simulink model "Test_Agent_Motor"  (R2018a)
settings: Solver=FixedStepAuto  StartTime=0.0  StopTime=inf  FixedStep=0.000001  RelTol=1e-3
(part 1 of 2)
settings Model: Creator=lenovo  LastModifiedBy=lenovo

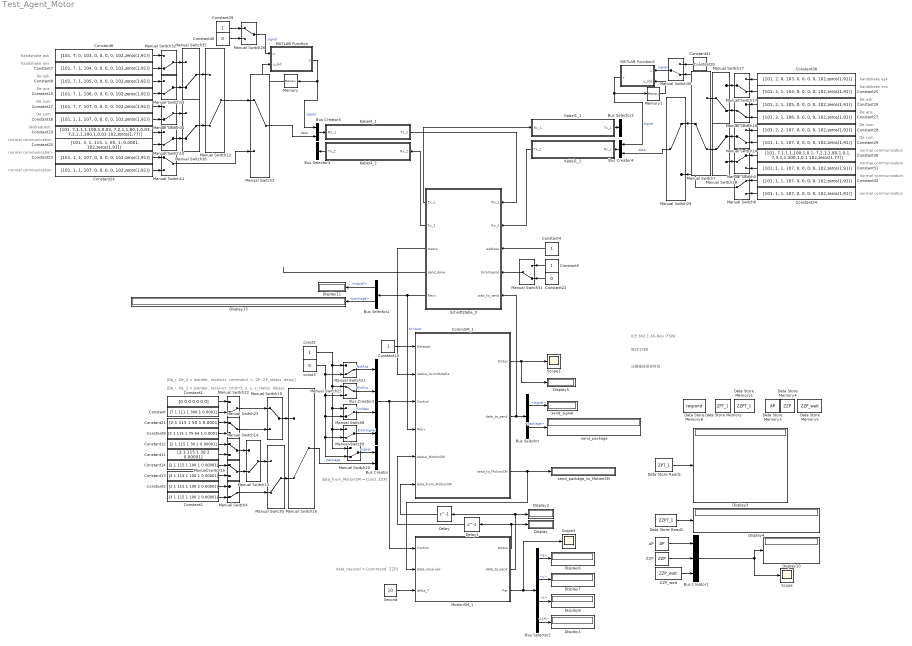
== system Test_Agent_Motor ==
  note: data_reeived = [command, ZZP]
  note: IEEE1588
  note: data_from_MotionSM = [cmd, ZZP]
  note: ICE 802.1 AS-Rev (TSN)
  note: [Da_i, De_i] = [sender, receiver, cmd=5, n, s, s_status, delay]
  note: [Da_i, De_i] = [sender, receiver, command, n, ZP, ZP_status, delay]
  note: 注意修改采样时间
  note: normal communication
  note: normal communication
  note: De ask
  note: handshake ans
  note: De sum
  note: normal communication
  note: handshake ask
  note: normal communication
  note: De sum
  note: normal communication
  note: De sum
  note: normal communication
  note: handshake ans
  note: handshake ask
  note: De ask
  note: Skillrequest
  note: De sum
  note: normal communication
  note: De ans
  note: De ans
  AP : DataStoreRead  DataStoreName=AP
  Bus Creator1 : BusCreator  Inputs=3
  Bus Creator : BusCreator  Inputs=2
  Bus Creator2 : BusCreator  Inputs=4
  Bus Creator4 : BusCreator  Inputs=2
  Bus Creator5 : BusCreator  Inputs=2
  Bus Selector : BusSelector  OutputSignals=signal,package
  Bus Selector1 : BusSelector  OutputSignals=a,v,s,AP
  Bus Selector2 : BusSelector  OutputSignals=signal,package
  Bus Selector3 : BusSelector  OutputSignals=signal,data
  Bus Selector4 : BusSelector  OutputSignals=signal,data
  CommSM_1 : Subsystem
  Constant : Constant  Value=[7 1 111 1 300 1 0.0001]  OutDataTypeStr=double
  Constant1 : Constant  Value=[0 0 0 0 0 0 0]  OutDataTypeStr=double
  Constant10 : Constant  Value=[101, 7, 1, 106, 0, 0, 0, 0, 102,zeros(1,91)]  OutDataTypeStr=double
  Constant11 : Constant  Value=[3 1 115 1 30 2 0.00001]  OutDataTypeStr=double
  Constant12 : Constant  Value=[2 1 115 1 30 2 0.00001]  OutDataTypeStr=double
  Constant13 : Constant  Value=[3 1 115 1 100 1 0.00001]  OutDataTypeStr=double
  Constant14 : Constant  Value=[2 1 115 1 100 1 0.00001]  OutDataTypeStr=double
  Constant15 : Constant  OutDataTypeStr=double
  Constant17 : Constant  Value=[101, 7, 7, 107, 0, 0, 0, 0, 102,zeros(1,91)]  OutDataTypeStr=double
  Constant{18,23..24,29,31..32,34} (7 alike) : Constant  Value=[101, 1, 1, 107, 0, 0, 0, 0, 102,zeros(1,91)]  OutDataTypeStr=double
  Constant19 : Constant  Value=[101, 7,1,1,1,100,1,0.03, 7,2,1,1,80,1,0.03, 7,3,1,1,300,1,0.03 102,zeros(1,77)]  OutDataTypeStr=double
  Constant2 : Constant  Value=[3 1 115 1 100 2 0.00001]  OutDataTypeStr=double
  Constant20 : Constant  Value=[101, 3, 1, 115, 1, 65, 1, 0.0001, 102,zeros(1,91)]  OutDataTypeStr=double
  Constant21 : Constant  Value=[2 1 115 1 50 1 0.0001]  OutDataTypeStr=double
  Constant22 : Constant  Value=0  OutDataTypeStr=boolean
  Constant25 : Constant  Value=[101, 2, 1, 104, 0, 0, 0, 0, 102,zeros(1,91)]  OutDataTypeStr=double
  Constant26 : Constant  Value=[101, 2, 1, 105, 0, 0, 0, 0, 102,zeros(1,91)]  OutDataTypeStr=double
  Constant27 : Constant  Value=[101, 2, 1, 106, 0, 0, 0, 0, 102,zeros(1,91)]  OutDataTypeStr=double
  Constant28 : Constant  Value=[101, 2, 2, 107, 0, 0, 0, 0, 102,zeros(1,91)]  OutDataTypeStr=double
  Constant3 : Constant  Value=[2 1 115 1 100 2 0.00001]  OutDataTypeStr=double
  Constant30 : Constant  Value=[101, 7,1,1,1,100,1,0.1, 7,2,1,1,80,1,0.1, 7,3,1,1,300,1,0.1 102,zeros(1,77)]  OutDataTypeStr=double
  Constant35 : Constant  Value=0  OutDataTypeStr=boolean
  Constant38 : Constant  Value=[101, 2, 0, 103, 0, 0, 0, 0, 102,zeros(1,91)]  OutDataTypeStr=double
  Constant39 : Constant  OutDataTypeStr=boolean
  Constant4 : Constant  OutDataTypeStr=double
  Constant40 : Constant  Value=0  OutDataTypeStr=boolean
  Constant41 : Constant  OutDataTypeStr=boolean
  Constant5 : Constant  OutDataTypeStr=boolean
  Constant6 : Constant  Value=[101, 7, 0, 103, 0, 0, 0, 0, 102,zeros(1,91)]  OutDataTypeStr=double
  Constant7 : Constant  Value=[101, 7, 1, 104, 0, 0, 0, 0, 102,zeros(1,91)]  OutDataTypeStr=double
  Constant8 : Constant  Value=[101, 7, 1, 105, 0, 0, 0, 0, 102,zeros(1,91)]  OutDataTypeStr=double
  Constant9 : Constant  Value=[3 1 115 1 75.64 1 0.0001]  OutDataTypeStr=double
  Data Store Memory : DataStoreMemory  DataStoreName=ZPT_1  ReadBeforeWriteMsg=warning  WriteAfterWriteMsg=warning  WriteAfterReadMsg=warning  InitialValue=zeros(10,3)  VectorParams1D=off  ShowAdditionalParam=off  OutDataTypeStr=double  Dimensions=[10,3]
  Data Store Memory1 : DataStoreMemory  DataStoreName=ZZPT_1  ReadBeforeWriteMsg=warning  WriteAfterWriteMsg=warning  WriteAfterReadMsg=warning  InitialValue=zeros(3,4)  VectorParams1D=off  ShowAdditionalParam=off  OutDataTypeStr=double  Dimensions=[3,4]
  Data Store Memory3 : DataStoreMemory  DataStoreName=AP  ReadBeforeWriteMsg=warning  WriteAfterWriteMsg=warning  WriteAfterReadMsg=warning  ShowAdditionalParam=off  OutMin=[0]  OutMax=[100]  OutDataTypeStr=double  Dimensions=1
  Data Store Memory4 : DataStoreMemory  DataStoreName=ZZP  ReadBeforeWriteMsg=warning  WriteAfterWriteMsg=warning  WriteAfterReadMsg=warning  ShowAdditionalParam=off  OutDataTypeStr=double  Dimensions=1
  Data Store Memory5 : DataStoreMemory  DataStoreName=ZZP_wait  ReadBeforeWriteMsg=warning  WriteAfterWriteMsg=warning  WriteAfterReadMsg=warning  ShowAdditionalParam=off  OutDataTypeStr=double  Dimensions=1
  Data Store Memory6 : DataStoreMemory  DataStoreName=respond  ReadBeforeWriteMsg=warning  WriteAfterWriteMsg=warning  WriteAfterReadMsg=warning  InitialValue=false  ShowAdditionalParam=off  OutDataTypeStr=boolean  Dimensions=1
  Data Store Read1 : DataStoreRead  DataStoreName=ZPT_1
  Data Store Read2 : DataStoreRead  DataStoreName=ZZPT_1
  Delay : Delay  DelayLength=1
  Delay1 : Delay  DelayLength=1
  Display{,1..8,10..11,13} (12 alike) : Display
      Display1 settings: Format=decimal (Stored Integer)
      Display10 settings: Format=decimal (Stored Integer)
      Display13 settings: Decimation=7
      Display8 settings: Format=decimal (Stored Integer)
  Kabel1_1 : Subsystem  TreatAsAtomicUnit=on
  Kabel1_2 : Subsystem  TreatAsAtomicUnit=on
  Kabel4_1 : Subsystem  TreatAsAtomicUnit=on
  Kabel4_2 : Subsystem  TreatAsAtomicUnit=on
  MATLAB Function : MATLAB Function  TreatAsAtomicUnit=on  SystemSampleTime=0.00001
  MATLAB Function1 : MATLAB Function  TreatAsAtomicUnit=on  SystemSampleTime=0.00001
  Manual Switch{4..5,7..10,12..13,16..18,20..22,24,27,30..36} (23 alike) : ManualSwitch  CurrentSetting=0
  Manual Switch{2..3,6,11,14..15,19,23,25..26,28..29} (12 alike) : ManualSwitch
  Memory : Memory  InitialCondition=false
  Memory1 : Memory  InitialCondition=false
  MotionSM_1 : Subsystem
  Schnittstelle_0 : Subsystem
  Scope : Scope
  Scope1 : Scope
  Scope3 : Scope
  Second : Constant  Value=10
  ZZP : DataStoreRead  DataStoreName=ZZP
  ZZP_wait : DataStoreRead  DataStoreName=ZZP_wait
  const2 : Constant  OutDataTypeStr=boolean
  const3 : Constant  Value=0  OutDataTypeStr=boolean
  send_package : Display
  send_package_to_MotionSM : Display
  send_signal : Display
  wires:
  Bus Selector1/2 -> Display7/1  "<v>"
  Manual Switch14/1 -> Manual Switch13/1
  Constant11/1 -> Manual Switch14/2
  Manual Switch9/1 -> Bus Creator2/4  "ErrorSignal"
  Manual Switch16/1 -> Bus Creator/2  "package"
  Manual Switch21/1 -> Bus Creator2/1  "NotAus"
  Bus Creator2/1 -> MotionSM_1/1(Control), CommSM_1/3(Control)
  CommSM_1/1(status) -> Display5/1, Scope1/1
  ZZP/1 -> Bus Creator1/2
  Manual Switch15/1 -> Manual Switch13/2
  Bus Selector1/3 -> Display8/1  "<s>"
  AP/1 -> Bus Creator1/1
  Manual Switch23/1 -> Manual Switch19/2
  Constant21/1 -> Manual Switch23/1
  Second/1 -> MotionSM_1/3(delta_T)
  ZZP_wait/1 -> Bus Creator1/3
  Manual Switch25/1 -> Bus Creator2/2  "EinAus"
  MotionSM_1/3(Par) -> Scope3/1, Bus Selector1/1
  Manual Switch4/1 -> Manual Switch5/2
  Manual Switch13/1 -> Manual Switch5/1
  Bus Creator1/1 -> Display10/1, Scope/1
  Constant12/1 -> Manual Switch14/1
  Manual Switch20/1 -> Bus Creator/1  "signal"
  MotionSM_1/2(data_to_send) -> Delay/1, Display2/1
  const2/1 -> Manual Switch20/1, Manual Switch9/1, Manual Switch8/1, Manual Switch25/1, Manual Switch21/1
  Delay/1 -> CommSM_1/6(data_from_MotionSM)
  Manual Switch19/1 -> Manual Switch16/1
  Constant13/1 -> Manual Switch15/2
  Constant1/1 -> Manual Switch22/1
  Bus Selector1/1 -> Display6/1  "<a>"
  CommSM_1/3(send_to_MotionSM) -> send_package_to_MotionSM/1, MotionSM_1/2(data_received)
  CommSM_1/2(data_to_send) -> Bus Selector/1, Schnittstelle_0/5(wait_to_send)
  Manual Switch8/1 -> Bus Creator2/3  "Richten"
  Manual Switch22/1 -> Manual Switch19/1
  Constant/1 -> Manual Switch22/2
  Constant9/1 -> Manual Switch23/2
  Bus Selector/2 -> send_package/1  "<package>"
  Bus Selector/1 -> send_signal/1  "<signal>"
  Data Store Read1/1 -> Display3/1
  MotionSM_1/1(status) -> Display/1, Delay1/1
  Delay1/1 -> CommSM_1/5(status_MotionSM)
  Constant2/1 -> Manual Switch4/2
  const3/1 -> Manual Switch20/2, Manual Switch9/2, Manual Switch8/2, Manual Switch25/2, Manual Switch21/2
  Constant3/1 -> Manual Switch4/1
  Manual Switch5/1 -> Manual Switch16/2
  Constant14/1 -> Manual Switch15/1
  Data Store Read2/1 -> Display4/1
  Bus Selector1/4 -> Display1/1  "<AP>"
  Constant35/1 -> Manual Switch30/2
  Manual Switch18/1 -> Manual Switch27/2
  Manual Switch30/1 -> MATLAB Function1/1(u)  "signal"
  Constant17/1 -> Manual Switch34/1
  Manual Switch32/1 -> Manual Switch35/1
  Constant41/1 -> Manual Switch30/1
  Manual Switch24/1 -> Manual Switch28/1
  Constant32/1 -> Manual Switch6/1
  Schnittstelle_0/1(Tx_1) -> Kabel1_1/1(Rx_1)
  Manual Switch26/1 -> MATLAB Function/1(u)  "signal"
  Manual Switch7/1 -> Manual Switch29/1
  Constant29/1 -> Manual Switch24/2
  Memory1/1 -> MATLAB Function1/2(u_old)
  Manual Switch6/1 -> Manual Switch29/2
  Constant6/1 -> Manual Switch32/1
  Manual Switch27/1 -> Manual Switch7/1
  Constant26/1 -> Manual Switch18/1
  Manual Switch17/1 -> Manual Switch27/1
  Constant27/1 -> Manual Switch18/2
  Constant7/1 -> Manual Switch32/2
  MATLAB Function/1(y) -> Bus Creator5/1, Memory/1  "signal"
  Schnittstelle_0/5(Recv) -> CommSM_1/4(Recv), Bus Selector2/1  "to Host"
  Memory/1 -> MATLAB Function/2(u_old)
  Manual Switch29/1 -> Bus Creator4/2  "data"
  Bus Creator4/1 -> Kabel1_2/1(Rx_2)
  Constant38/1 -> Manual Switch17/1
  Constant24/1 -> Manual Switch11/2
  Manual Switch34/1 -> Manual Switch36/1
  Constant10/1 -> Manual Switch33/2
  Constant23/1 -> Manual Switch11/1
  Manual Switch28/1 -> Manual Switch7/2
  Constant5/1 -> Manual Switch31/1
  Manual Switch36/1 -> Manual Switch12/2
  Constant19/1 -> Manual Switch10/1
  Manual Switch3/1 -> Manual Switch28/2
  Constant30/1 -> Manual Switch3/1
  Constant20/1 -> Manual Switch10/2
  Schnittstelle_0/3(status) -> CommSM_1/2(status_Schnittstelle)
  Bus Creator5/1 -> Kabel4_1/1(Rx_1)
  Manual Switch12/1 -> Manual Switch2/1
  Schnittstelle_0/2(Tx_2) -> Kabel4_2/1(Rx_2)
  Manual Switch2/1 -> Bus Creator5/2  "data"
  Constant39/1 -> Manual Switch26/1
  Constant18/1 -> Manual Switch34/2
  Manual Switch33/1 -> Manual Switch35/2
  Manual Switch11/1 -> Manual Switch2/2
  Kabel1_2/1(Tx_2) -> Schnittstelle_0/2(Rx_2)
  MATLAB Function1/1(y) -> Bus Creator4/1, Memory1/1  "signal"
  Constant22/1 -> Manual Switch31/2
  Kabel4_2/1(Tx_2) -> Bus Selector4/1
  Manual Switch31/1 -> Schnittstelle_0/4(ErrorSignal)
  Constant31/1 -> Manual Switch3/2
  Constant8/1 -> Manual Switch33/1
  Kabel1_1/1(Tx_1) -> Bus Selector3/1
  Bus Selector2/2 -> Display13/1  "<package>"
  Bus Selector2/1 -> Display11/1  "<signal>"
  Constant40/1 -> Manual Switch26/2
  Manual Switch35/1 -> Manual Switch12/1
  Manual Switch10/1 -> Manual Switch36/2
  Constant34/1 -> Manual Switch6/2
  Kabel4_1/1(Tx_1) -> Schnittstelle_0/1(Rx_1)
  Constant25/1 -> Manual Switch17/2
  Constant28/1 -> Manual Switch24/1
  Constant4/1 -> Schnittstelle_0/3(address)
  Constant15/1 -> CommSM_1/1(Adresse)
  Schnittstelle_0/4(send_done) -> ?

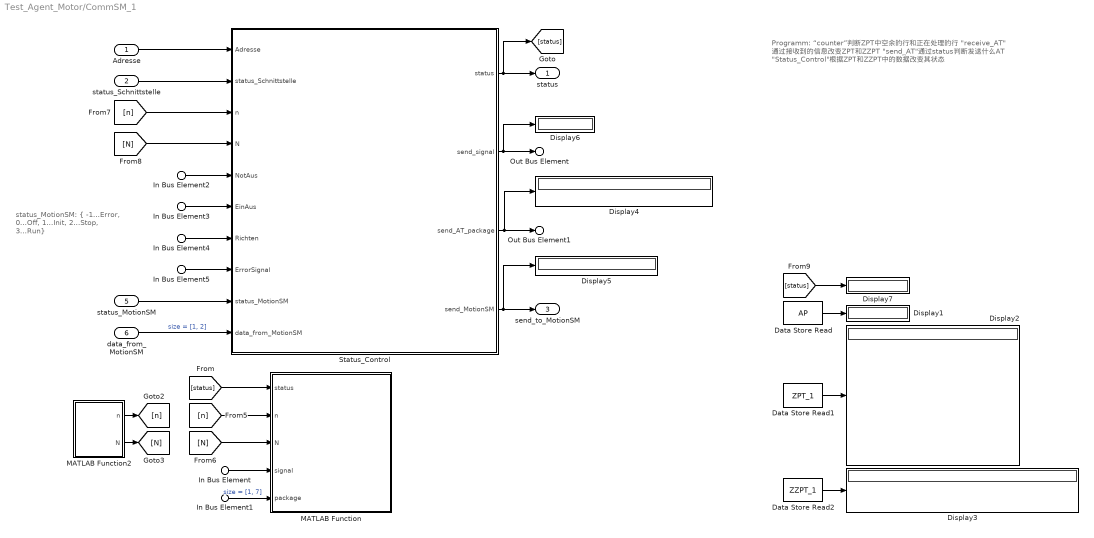
== system Test_Agent_Motor/CommSM_1 ==
  note: Programm:
      | “counter”判断ZPT中空余的行和正在处理的行
      | "receive_AT" 通过接收到的信息改变ZPT和ZZPT
      | "send_AT"通过status判断发送什么AT
      | "Status_Control"根据ZPT和ZZPT中的数据改变其状态
  note: status_MotionSM: {
      | -1...Error,
      | 0...Off,
      | 1...Init,
      | 2...Stop,
      | 3...Run}
  Adresse : Inport  OutDataTypeStr=double  PortDimensions=1
  status_Schnittstelle : Inport  Port=2  OutDataTypeStr=double  PortDimensions=1
  In Bus Element2 : Inport  Port=3  PortName=Control  Element=NotAus
  In Bus Element3 : Inport  Port=3  PortName=Control  Element=EinAus
  In Bus Element4 : Inport  Port=3  PortName=Control  Element=Richten
  In Bus Element5 : Inport  Port=3  PortName=Control  Element=ErrorSignal
  In Bus Element : Inport  Port=4  PortName=Recv  Element=signal
  In Bus Element1 : Inport  Port=4  PortName=Recv  Element=package
  status_MotionSM : Inport  Port=5  OutDataTypeStr=double  PortDimensions=1
  data_from_MotionSM : Inport  Port=6  OutDataTypeStr=double  PortDimensions=2
  Data Store Read : DataStoreRead  DataStoreName=AP
  Data Store Read1 : DataStoreRead  DataStoreName=ZPT_1
  Data Store Read2 : DataStoreRead  DataStoreName=ZZPT_1
  Display{1..7} (7 alike) : Display
  MATLAB Function : MATLAB Function  TreatAsAtomicUnit=on
  MATLAB Function2 : MATLAB Function  TreatAsAtomicUnit=on
  Status_Control : Stateflow chart  TreatAsAtomicUnit=on
  status : Outport  OutDataTypeStr=double  PortDimensions=1
  Out Bus Element : Outport  Port=2  PortName=data_to_send  Element=signal
  Out Bus Element1 : Outport  Port=2  PortName=data_to_send  Element=package
  send_to_MotionSM : Outport  Port=3
  wires:
  In Bus Element2/1 -> Status_Control/5(NotAus)
  In Bus Element3/1 -> Status_Control/6(EinAus)
  In Bus Element4/1 -> Status_Control/7(Richten)
  In Bus Element5/1 -> Status_Control/8(ErrorSignal)
  status_Schnittstelle/1 -> Status_Control/2(status_Schnittstelle)
  In Bus Element/1 -> MATLAB Function/4(signal)
  In Bus Element1/1 -> MATLAB Function/5(package)  "size = [1, 7]"
  data_from_MotionSM/1 -> Status_Control/10(data_from_MotionSM)  "size = [1, 2]"
  status_MotionSM/1 -> Status_Control/9(status_MotionSM)
  Adresse/1 -> Status_Control/1(Adresse)
  Status_Control/1(status) -> [status], status/1
  Status_Control/3(send_AT_package) -> Out Bus Element1/1, Display4/1
  Status_Control/4(send_MotionSM) -> send_to_MotionSM/1, Display5/1
  Status_Control/2(send_signal) -> Out Bus Element/1, Display6/1
  Data Store Read/1 -> Display1/1
  Data Store Read1/1 -> Display2/1
  Data Store Read2/1 -> Display3/1
  [status] -> MATLAB Function/1(status)
  MATLAB Function2/1(n) -> [n]
  MATLAB Function2/2(N) -> [N]
  [N] -> MATLAB Function/3(N)
  [n] -> MATLAB Function/2(n)
  [n] -> Status_Control/3(n)
  [N] -> Status_Control/4(N)
  [status] -> Display7/1

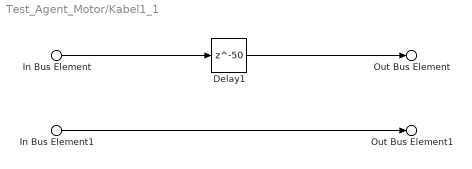
== system Test_Agent_Motor/Kabel1_1 ==
  In Bus Element : Inport  PortName=Rx_1  Element=signal
  In Bus Element1 : Inport  PortName=Rx_1  Element=data
  Delay1 : Delay  DelayLength=50
  Out Bus Element : Outport  PortName=Tx_1  Element=signal
  Out Bus Element1 : Outport  PortName=Tx_1  Element=data
  wires:
  In Bus Element/1 -> Delay1/1
  Delay1/1 -> Out Bus Element/1
  In Bus Element1/1 -> Out Bus Element1/1

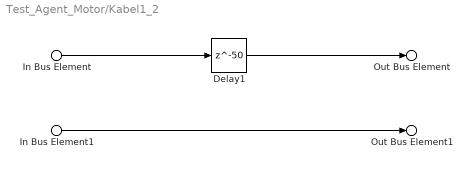
== system Test_Agent_Motor/Kabel1_2 ==
  In Bus Element : Inport  PortName=Rx_2  Element=signal
  In Bus Element1 : Inport  PortName=Rx_2  Element=data
  Delay1 : Delay  DelayLength=50
  Out Bus Element : Outport  PortName=Tx_2  Element=signal
  Out Bus Element1 : Outport  PortName=Tx_2  Element=data
  wires:
  In Bus Element/1 -> Delay1/1
  Delay1/1 -> Out Bus Element/1
  In Bus Element1/1 -> Out Bus Element1/1

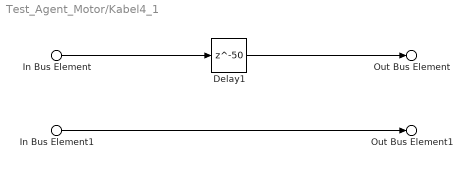
== system Test_Agent_Motor/Kabel4_1 ==
  In Bus Element : Inport  PortName=Rx_1  Element=signal
  In Bus Element1 : Inport  PortName=Rx_1  Element=data
  Delay1 : Delay  DelayLength=50
  Out Bus Element : Outport  PortName=Tx_1  Element=signal
  Out Bus Element1 : Outport  PortName=Tx_1  Element=data
  wires:
  In Bus Element/1 -> Delay1/1
  Delay1/1 -> Out Bus Element/1
  In Bus Element1/1 -> Out Bus Element1/1

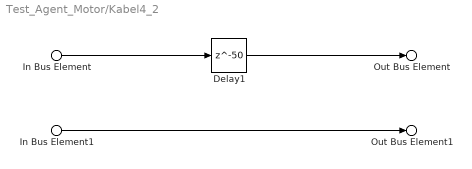
== system Test_Agent_Motor/Kabel4_2 ==
  In Bus Element : Inport  PortName=Rx_2  Element=signal
  In Bus Element1 : Inport  PortName=Rx_2  Element=data
  Delay1 : Delay  DelayLength=50
  Out Bus Element : Outport  PortName=Tx_2  Element=signal
  Out Bus Element1 : Outport  PortName=Tx_2  Element=data
  wires:
  In Bus Element/1 -> Delay1/1
  Delay1/1 -> Out Bus Element/1
  In Bus Element1/1 -> Out Bus Element1/1

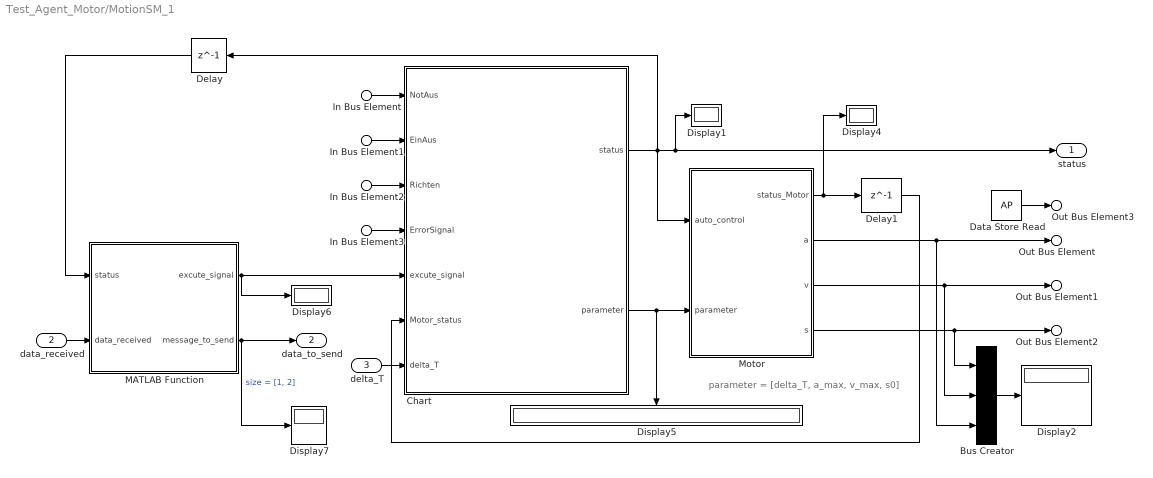
== system Test_Agent_Motor/MotionSM_1 ==
  note: parameter = [delta_T, a_max, v_max, s0]
  In Bus Element : Inport  PortName=Control  Element=NotAus
  In Bus Element1 : Inport  PortName=Control  Element=EinAus
  In Bus Element2 : Inport  PortName=Control  Element=Richten
  In Bus Element3 : Inport  PortName=Control  Element=ErrorSignal
  data_received : Inport  Port=2  OutDataTypeStr=double  PortDimensions=2
  delta_T : Inport  Port=3
  Bus Creator : BusCreator  Inputs=3
  Chart : Stateflow chart  TreatAsAtomicUnit=on
  Data Store Read : DataStoreRead  DataStoreName=AP
  Delay : Delay  DelayLength=1
  Delay1 : Delay  DelayLength=1
  Display{1..2,4..7} (6 alike) : Display
  MATLAB Function : MATLAB Function  TreatAsAtomicUnit=on
  Motor : Subsystem
  status : Outport
  data_to_send : Outport  Port=2  OutDataTypeStr=double  PortDimensions=2
  Out Bus Element : Outport  Port=3  PortName=Par  Element=a
  Out Bus Element1 : Outport  Port=3  PortName=Par  Element=v
  Out Bus Element2 : Outport  Port=3  PortName=Par  Element=s
  Out Bus Element3 : Outport  Port=3  PortName=Par  Element=AP
  wires:
  Chart/1(status) -> Motor/1(auto_control), Delay/1, Display1/1, status/1
  In Bus Element1/1 -> Chart/2(EinAus)
  In Bus Element/1 -> Chart/1(NotAus)
  In Bus Element2/1 -> Chart/3(Richten)
  In Bus Element3/1 -> Chart/4(ErrorSignal)
  Motor/1(status_Motor) -> Display4/1, Delay1/1
  data_received/1 -> MATLAB Function/2(data_received)
  Delay1/1 -> Chart/6(Motor_status)
  MATLAB Function/1(excute_signal) -> Display6/1, Chart/5(excute_signal)
  MATLAB Function/2(message_to_send) -> data_to_send/1, Display7/1  "size = [1, 2]"
  delta_T/1 -> Chart/7(delta_T)
  Motor/2(a) -> Bus Creator/3, Out Bus Element/1
  Motor/3(v) -> Bus Creator/2, Out Bus Element1/1
  Motor/4(s) -> Bus Creator/1, Out Bus Element2/1
  Chart/2(parameter) -> Motor/2(parameter), Display5/1
  Delay/1 -> MATLAB Function/1(status)
  Data Store Read/1 -> Out Bus Element3/1
  Bus Creator/1 -> Display2/1

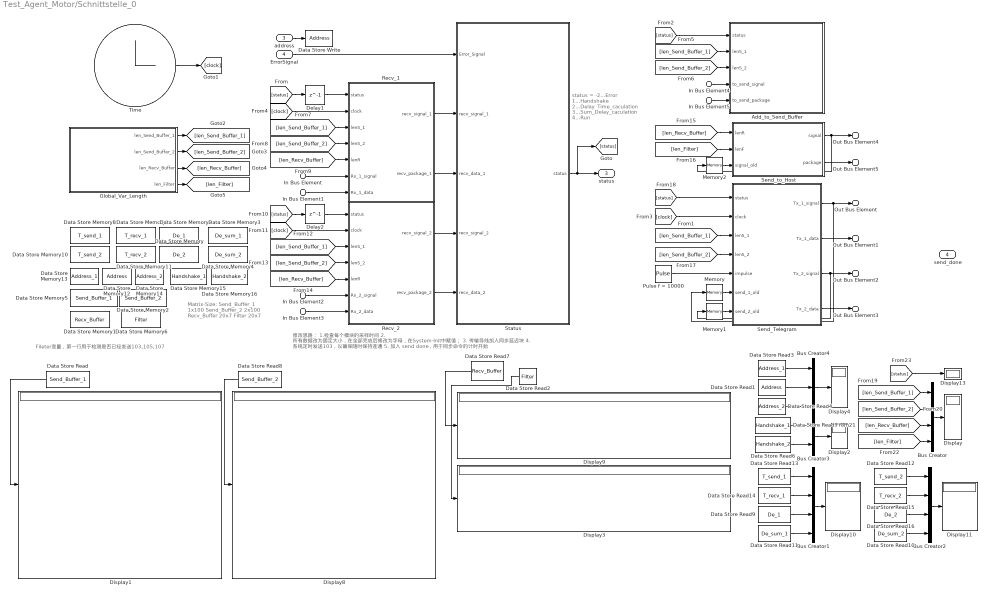
== system Test_Agent_Motor/Schnittstelle_0 ==
  note: Fileter变量，第一行用于检测是否已经发送103,105,107
  note: 修改思路：
      | 1.检查每个模块的采样时间
      | 2. 所有数据改为固定大小，在全部完成后修改为字母，在System-Init中赋值；
      | 3. 传输导线加入同步延迟块
      | 4. 系统定时发送103，以确保随时保持连通
      | 5. 加入 send done，用于同步命令的计时开始
  note: status =
      | -2...Error
      |  1...Handshake
      |  2...Delay_Time_caculation
      |  3...Sum_Delay_caculation
      |  4...Run
  note: Matrix-Size:
      | Send_Buffer_1	1x100
      | Send_Buffer_2	2x100
      | Recv_Buffer		20x7
      | Filter			20x7
  In Bus Element : Inport  PortName=Rx_1  Element=signal
  In Bus Element1 : Inport  PortName=Rx_1  Element=data
  In Bus Element2 : Inport  Port=2  PortName=Rx_2  Element=signal
  In Bus Element3 : Inport  Port=2  PortName=Rx_2  Element=data
  address : Inport  Port=3
  ErrorSignal : Inport  Port=4
  In Bus Element4 : Inport  Port=5  PortName=wait_to_send  Element=signal
  In Bus Element5 : Inport  Port=5  PortName=wait_to_send  Element=package
  Add_to_Send_Buffer : MATLAB Function  TreatAsAtomicUnit=on  SystemSampleTime=0.00001
  Bus Creator : BusCreator  Inputs=4
  Bus Creator1 : BusCreator  Inputs=4
  Bus Creator2 : BusCreator  Inputs=4
  Bus Creator3 : BusCreator  Inputs=2
  Bus Creator4 : BusCreator  Inputs=3
  Data Store Memory : DataStoreMemory  DataStoreName=De_2  ReadBeforeWriteMsg=warning  WriteAfterWriteMsg=warning  WriteAfterReadMsg=warning  ShowAdditionalParam=off  OutDataTypeStr=double  Dimensions=1
  Data Store Memory1 : DataStoreMemory  DataStoreName=Recv_Buffer  ReadBeforeWriteMsg=warning  WriteAfterWriteMsg=warning  WriteAfterReadMsg=warning  InitialValue=zeros(20,7)  VectorParams1D=off  ShowAdditionalParam=off  OutDataTypeStr=double  Dimensions=[20,7]
  Data Store Memory10 : DataStoreMemory  DataStoreName=T_send_2  ReadBeforeWriteMsg=warning  WriteAfterWriteMsg=warning  WriteAfterReadMsg=warning  ShowAdditionalParam=off  OutDataTypeStr=double  Dimensions=1
  Data Store Memory11 : DataStoreMemory  DataStoreName=T_recv_2  ReadBeforeWriteMsg=warning  WriteAfterWriteMsg=warning  WriteAfterReadMsg=warning  ShowAdditionalParam=off  OutDataTypeStr=double  Dimensions=1
  Data Store Memory12 : DataStoreMemory  DataStoreName=Address  ReadBeforeWriteMsg=warning  WriteAfterWriteMsg=warning  WriteAfterReadMsg=warning  ShowAdditionalParam=off  OutDataTypeStr=double  Dimensions=1
  Data Store Memory13 : DataStoreMemory  DataStoreName=Address_1  ReadBeforeWriteMsg=warning  WriteAfterWriteMsg=warning  WriteAfterReadMsg=warning  ShowAdditionalParam=off  OutDataTypeStr=double  Dimensions=1
  Data Store Memory14 : DataStoreMemory  DataStoreName=Address_2  ReadBeforeWriteMsg=warning  WriteAfterWriteMsg=warning  WriteAfterReadMsg=warning  ShowAdditionalParam=off  OutDataTypeStr=double  Dimensions=1
  Data Store Memory15 : DataStoreMemory  DataStoreName=Handshake_1  ReadBeforeWriteMsg=warning  WriteAfterWriteMsg=warning  WriteAfterReadMsg=warning  InitialValue=false  ShowAdditionalParam=off  OutDataTypeStr=boolean
  Data Store Memory16 : DataStoreMemory  DataStoreName=Handshake_2  ReadBeforeWriteMsg=warning  WriteAfterWriteMsg=warning  WriteAfterReadMsg=warning  InitialValue=false  ShowAdditionalParam=off  OutDataTypeStr=boolean
  Data Store Memory2 : DataStoreMemory  DataStoreName=Send_Buffer_2  ReadBeforeWriteMsg=warning  WriteAfterWriteMsg=warning  WriteAfterReadMsg=warning  InitialValue=[101, 102, zeros(1,98)]  VectorParams1D=off  ShowAdditionalParam=off  OutDataTypeStr=double  Dimensions=[1,100]
  Data Store Memory3 : DataStoreMemory  DataStoreName=De_sum_1  ReadBeforeWriteMsg=warning  WriteAfterWriteMsg=warning  WriteAfterReadMsg=warning  ShowAdditionalParam=off  OutDataTypeStr=double  Dimensions=1
  Data Store Memory4 : DataStoreMemory  DataStoreName=De_sum_2  ReadBeforeWriteMsg=warning  WriteAfterWriteMsg=warning  WriteAfterReadMsg=warning  ShowAdditionalParam=off  OutDataTypeStr=double  Dimensions=1
  Data Store Memory5 : DataStoreMemory  DataStoreName=Send_Buffer_1  ReadBeforeWriteMsg=warning  WriteAfterWriteMsg=warning  WriteAfterReadMsg=warning  InitialValue=[101, 102, zeros(1,98)]  VectorParams1D=off  ShowAdditionalParam=off  OutDataTypeStr=double  Dimensions=[1,100]
  Data Store Memory6 : DataStoreMemory  DataStoreName=Filter  ReadBeforeWriteMsg=warning  WriteAfterWriteMsg=warning  WriteAfterReadMsg=warning  InitialValue=zeros(20,7)  VectorParams1D=off  ShowAdditionalParam=off  OutDataTypeStr=double  Dimensions=[20,7]
  Data Store Memory7 : DataStoreMemory  DataStoreName=De_1  ReadBeforeWriteMsg=warning  WriteAfterWriteMsg=warning  WriteAfterReadMsg=warning  ShowAdditionalParam=off  OutDataTypeStr=double  Dimensions=1
  Data Store Memory8 : DataStoreMemory  DataStoreName=T_send_1  ReadBeforeWriteMsg=warning  WriteAfterWriteMsg=warning  WriteAfterReadMsg=warning  ShowAdditionalParam=off  OutDataTypeStr=double  Dimensions=1
  Data Store Memory9 : DataStoreMemory  DataStoreName=T_recv_1  ReadBeforeWriteMsg=warning  WriteAfterWriteMsg=warning  WriteAfterReadMsg=warning  ShowAdditionalParam=off  OutDataTypeStr=double  Dimensions=1
  Data Store Read : DataStoreRead  DataStoreName=Send_Buffer_1
  Data Store Read1 : DataStoreRead  DataStoreName=Address
  Data Store Read10 : DataStoreRead  DataStoreName=De_sum_2
  Data Store Read11 : DataStoreRead  DataStoreName=De_sum_1
  Data Store Read12 : DataStoreRead  DataStoreName=T_send_2
  Data Store Read13 : DataStoreRead  DataStoreName=T_send_1
  Data Store Read14 : DataStoreRead  DataStoreName=T_recv_1
  Data Store Read15 : DataStoreRead  DataStoreName=T_recv_2
  Data Store Read16 : DataStoreRead  DataStoreName=De_2
  Data Store Read2 : DataStoreRead  DataStoreName=Filter
  Data Store Read3 : DataStoreRead  DataStoreName=Address_1
  Data Store Read4 : DataStoreRead  DataStoreName=Address_2
  Data Store Read5 : DataStoreRead  DataStoreName=Handshake_1
  Data Store Read6 : DataStoreRead  DataStoreName=Handshake_2
  Data Store Read7 : DataStoreRead  DataStoreName=Recv_Buffer
  Data Store Read8 : DataStoreRead  DataStoreName=Send_Buffer_2
  Data Store Read9 : DataStoreRead  DataStoreName=De_1
  Data Store Write : DataStoreWrite  DataStoreName=Address
  Delay1 : Delay  DelayLength=1
  Delay2 : Delay  DelayLength=1
  Display{,1..4,8..11,13} (10 alike) : Display
  Global_Var_Length : MATLAB Function  TreatAsAtomicUnit=on
  Memory : Memory  InitialCondition=false
  Memory1 : Memory  InitialCondition=false
  Memory2 : Memory  InitialCondition=false
  Pulse f = 10000 : DiscretePulseGenerator  PulseType=Time based  Amplitude=true  Period=1/1000  PulseWidth=30
  Recv_1 : MATLAB Function  TreatAsAtomicUnit=on  SystemSampleTime=0.00001
  Recv_2 : MATLAB Function  TreatAsAtomicUnit=on  SystemSampleTime=0.00001
  Send_Telegram : MATLAB Function  TreatAsAtomicUnit=on  SystemSampleTime=0.00001
  Send_to_Host : MATLAB Function  TreatAsAtomicUnit=on  SystemSampleTime=0.00001
  Status : Stateflow chart  TreatAsAtomicUnit=on  SystemSampleTime=0.0000001
  Time : Clock
  Out Bus Element : Outport  PortName=Tx_1  Element=signal
  Out Bus Element1 : Outport  PortName=Tx_1  Element=data
  Out Bus Element2 : Outport  Port=2  PortName=Tx_2  Element=signal
  Out Bus Element3 : Outport  Port=2  PortName=Tx_2  Element=data
  status : Outport  Port=3
  send_done : Outport  Port=4
  Out Bus Element4 : Outport  Port=5  PortName=Recv  Element=signal
  Out Bus Element5 : Outport  Port=5  PortName=Recv  Element=package
  wires:
  ErrorSignal/1 -> Status/1(Error_Signal)
  Status/1(status) -> [status], status/1
  Pulse f = 10000/1 -> Send_Telegram/5(impulse)
  In Bus Element1/1 -> Recv_1/7(Rx_1_data)
  In Bus Element/1 -> Recv_1/6(Rx_1_signal)
  Send_Telegram/1(Tx_1_signal) -> Memory/1, Out Bus Element/1
  Send_Telegram/3(Tx_2_signal) -> Memory1/1, Out Bus Element2/1
  Memory1/1 -> Send_Telegram/7(send_2_old)
  Memory/1 -> Send_Telegram/6(send_1_old)
  [status] -> Delay1/1
  Time/1 -> [clock]
  [clock] -> Recv_1/2(clock)
  Send_to_Host/1(signal) -> Out Bus Element4/1, Memory2/1
  address/1 -> Data Store Write/1
  Global_Var_Length/1(len_Send_Buffer_1) -> [len_Send_Buffer_1]
  Global_Var_Length/2(len_Send_Buffer_2) -> [len_Send_Buffer_2]
  Global_Var_Length/3(len_Recv_Buffer) -> [len_Recv_Buffer]
  Global_Var_Length/4(len_Filter) -> [len_Filter]
  [len_Send_Buffer_1] -> Recv_1/3(lenS_1)
  [len_Send_Buffer_2] -> Recv_1/4(lenS_2)
  [len_Recv_Buffer] -> Recv_1/5(lenR)
  In Bus Element2/1 -> Recv_2/6(Rx_2_signal)
  In Bus Element3/1 -> Recv_2/7(Rx_2_data)
  [status] -> Delay2/1
  [len_Recv_Buffer] -> Recv_2/5(lenR)
  [len_Send_Buffer_1] -> Recv_2/3(lenS_1)
  [clock] -> Recv_2/2(clock)
  [len_Send_Buffer_2] -> Recv_2/4(lenS_2)
  Delay1/1 -> Recv_1/1(status)
  Delay2/1 -> Recv_2/1(status)
  Recv_1/1(recv_signal_1) -> Status/2(recv_signal_1)
  Recv_1/2(recv_package_1) -> Status/3(recv_data_1)
  Recv_2/1(recv_signal_2) -> Status/4(recv_signal_2)
  Recv_2/2(recv_package_2) -> Status/5(recv_data_2)
  [len_Recv_Buffer] -> Send_to_Host/1(lenR)
  [len_Filter] -> Send_to_Host/2(lenF)
  Send_Telegram/4(Tx_2_data) -> Out Bus Element3/1
  [len_Send_Buffer_1] -> Send_Telegram/3(lenS_1)
  [len_Send_Buffer_2] -> Send_Telegram/4(lenS_2)
  [clock] -> Send_Telegram/2(clock)
  [status] -> Send_Telegram/1(status)
  Send_Telegram/2(Tx_1_data) -> Out Bus Element1/1
  [len_Send_Buffer_1] -> Add_to_Send_Buffer/2(lenS_1)
  [len_Send_Buffer_2] -> Add_to_Send_Buffer/3(lenS_2)
  In Bus Element4/1 -> Add_to_Send_Buffer/4(to_send_signal)
  In Bus Element5/1 -> Add_to_Send_Buffer/5(to_send_package)
  [status] -> Add_to_Send_Buffer/1(status)
  Memory2/1 -> Send_to_Host/3(signal_old)
  Bus Creator/1 -> Display/1
  [len_Send_Buffer_1] -> Bus Creator/1
  [len_Send_Buffer_2] -> Bus Creator/2
  [len_Recv_Buffer] -> Bus Creator/3
  [len_Filter] -> Bus Creator/4
  Data Store Read/1 -> Display1/1
  Data Store Read2/1 -> Display3/1
  Data Store Read8/1 -> Display8/1
  Data Store Read7/1 -> Display9/1
  Data Store Read13/1 -> Bus Creator1/1
  Data Store Read14/1 -> Bus Creator1/2
  Data Store Read11/1 -> Bus Creator1/4
  Data Store Read9/1 -> Bus Creator1/3
  Bus Creator1/1 -> Display10/1
  Data Store Read12/1 -> Bus Creator2/1
  Data Store Read15/1 -> Bus Creator2/2
  Bus Creator2/1 -> Display11/1
  Data Store Read16/1 -> Bus Creator2/3
  Data Store Read10/1 -> Bus Creator2/4
  [status] -> Display13/1
  Send_to_Host/2(package) -> Out Bus Element5/1
  Data Store Read5/1 -> Bus Creator3/1
  Data Store Read6/1 -> Bus Creator3/2
  Data Store Read4/1 -> Bus Creator4/3
  Data Store Read1/1 -> Bus Creator4/2
  Data Store Read3/1 -> Bus Creator4/1
  Bus Creator3/1 -> Display2/1
  Bus Creator4/1 -> Display4/1

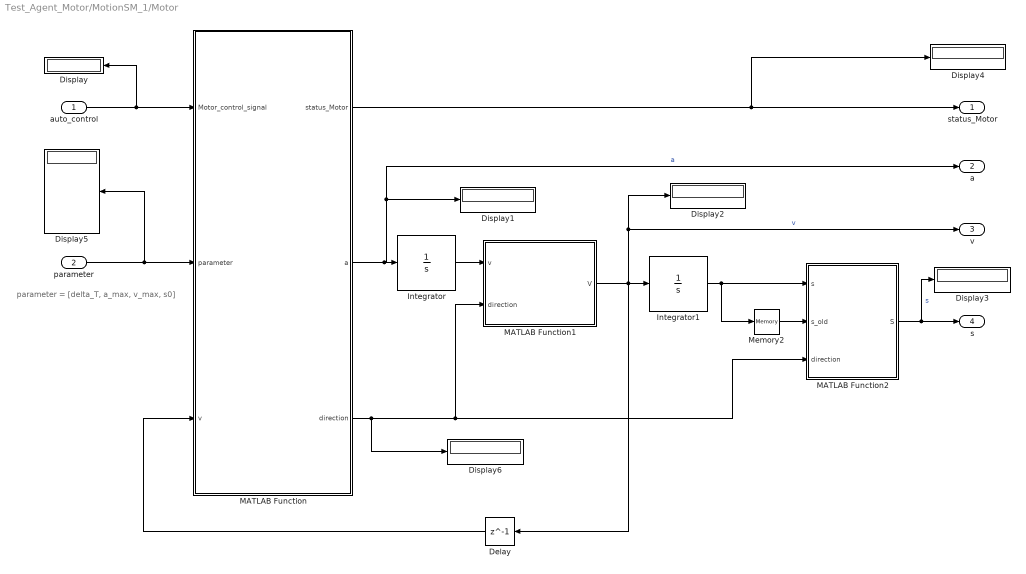
== system Test_Agent_Motor/MotionSM_1/Motor ==
  note: parameter = [delta_T, a_max, v_max, s0]
  auto_control : Inport
  parameter : Inport  Port=2
  Delay : Delay  DelayLength=1
  Display{,1..6} (7 alike) : Display
  Integrator : Integrator
  Integrator1 : Integrator
  MATLAB Function : MATLAB Function  TreatAsAtomicUnit=on
  MATLAB Function1 : MATLAB Function  TreatAsAtomicUnit=on
  MATLAB Function2 : MATLAB Function  TreatAsAtomicUnit=on
  Memory2 : Memory
  status_Motor : Outport
  a : Outport  Port=2
  v : Outport  Port=3
  s : Outport  Port=4
  wires:
  Integrator/1 -> MATLAB Function1/1(v)
  Integrator1/1 -> MATLAB Function2/1(s), Memory2/1
  auto_control/1 -> Display/1, MATLAB Function/1(Motor_control_signal)
  MATLAB Function/1(status_Motor) -> Display4/1, status_Motor/1
  parameter/1 -> Display5/1, MATLAB Function/2(parameter)
  MATLAB Function/2(a) -> a/1, Display1/1, Integrator/1  "a"
  MATLAB Function1/1(V) -> Display2/1, v/1, Delay/1, Integrator1/1  "v"
  MATLAB Function/3(direction) -> MATLAB Function1/2(direction), MATLAB Function2/3(direction), Display6/1
  MATLAB Function2/1(S) -> Display3/1, s/1  "s"
  Memory2/1 -> MATLAB Function2/2(s_old)
  Delay/1 -> MATLAB Function/3(v)

== matlab function Test_Agent_Motor/MotionSM_1/MATLAB Function ==
  data: status input double size=1; excute_signal output boolean size=1; message_to_send output double size=2; data_received input double size=2; ZZP_wait data_store_memory size=1; AP data_store_memory; ZZP data_store_memory
%data_received / message_to_send = [cmd, ZZP]
%cmd:  1...setP, 2...getP, 3...excP

function [excute_signal, message_to_send] = message_analysis(status, data_received)

global ZZP_wait
global AP
global ZZP

excute_signal = false;

cmd = data_received(1);
message_to_send = [0, 0]';

switch cmd
    case 1      % setP
        excute_signal = false;
        if ((status >= 1) && (status <= 3))
            ZZP_wait = data_received(2);
            message_to_send = [2, ZZP_wait]';   % getP
        end
        
    case 3      % excP
        excute_signal = true;
        if ((ZZP == AP) && (status == 2) && (ZZP~=ZZP_wait))
            ZZP = ZZP_wait;
        end
end
end

== matlab function Test_Agent_Motor/MotionSM_1/Motor/MATLAB Function ==
  settings: updateMethod=DISCRETE
  data: status_Motor output boolean size=1; Motor_control_signal input double size=1; parameter input double size=4; v input double size=1; a output double size=1; direction output double size=1; AP data_store_memory; ZZP data_store_memory
function [status_Motor, a, direction]= Motor(Motor_control_signal, parameter, v)

%delta_T = parameter(1);
a_max = abs(parameter(2));
v_max = abs(parameter(3));
s0 = parameter(4);
direction = 0;
a = 0;

s_a = 0.5 * v_max * v_max / a_max;
a_bremsen = 100000;     % 100 m/s^2

global AP
global ZZP

switch Motor_control_signal
    case {-1, 0}            %Error & Off
        if v > 0
            a = -a_bremsen;
            direction = 1;
        elseif v < 0
            a = a_bremsen;
            direction = -1;
        else
            a = 0;
            direction = 0;
        end
             
    case 1                  %Init
        if (AP > 0)
            direction = s0;
            if ((ZZP - AP) < (-s_a)) && (v > (-v_max))
                a = -a_max;
            elseif ((ZZP - AP) >= (-s_a)) && (ZZP < AP) && (v < 0)
                a = a_max;
            else
                a = 0;
            end
        else
            a = 0;
            AP = 0;
        end
        
    case 2                  %Stop
        if (v > 0)
            a = -a_max;
            direction = 1;
        elseif (v < 0)
            a = a_max;
            direction = -1;
        else
            a = 0;
            direction = 0;
        end
        
    case 3                  %run
        direction = s0;
        if (s0 > 0)   %forward
            %v_control(2) = s0;
            if ((ZZP - AP) > s_a) && (v < v_max)
                a = a_max;
            elseif ((ZZP - AP) <= s_a) && (ZZP > AP) && (v > 0)
                a = -a_max;
            else
                a = 0;
            end
        end
        if (s0 < 0)    %backward
            if ((ZZP - AP) < (-s_a)) && (v > (-v_max))
                a = -a_max;
            elseif ((ZZP - AP) >= (-s_a)) && (ZZP < AP) && (v < 0)
                a = a_max;
            else
                a = 0;
            end
        end
end
        
%status_Motor: false...Stopped, true...Running
if (a == 0) && (v == 0)
    status_Motor = false;
else
    status_Motor = true;
end

end

== stateflow chart Test_Agent_Motor/MotionSM_1/Chart ==
  state Off
    entry: status=0;
  state Init
    entry: status=1; parameter=Par_1(delta_T);
  state On
    state Stop
      entry: status=2;
    state Run
      entry: status=3;
    (default) -> Stop
    Stop -> Run : [excute_signal==1 && ZZP~=AP && Motor_status == 0]
        | {parameter=Par(delta_T)}
    Run -> Stop : [ZZP==AP && ~Motor_status]
  state Error
    entry: status=-1;
  (default) -> Off
  Init -> Off [order 1] : [~EinAus]
  Off -> Init [order 2] : [EinAus && ~ NotAus]{parameter=[delta_T,0,0,0]'}
  Init -> Error [order 2] : [Motor_status==-1 || NotAus || ErrorSignal]
  Off -> Error [order 1] : [EinAus && (ErrorSignal || NotAus)]
  Error -> Off [order 1] : [~EinAus]
  On -> Off [order 1] : [~EinAus]
  Error -> Init [order 2] : [Richten]{parameter=[delta_T,0,0,0]'}
  Init -> On [order 3] : [AP==0]{parameter=[delta_T,0,0,0]'}
  On -> Error [order 2] : [Motor_status==-1 || NotAus || ErrorSignal]
  data: par function_output double size=4; delta_t function_input double size=1; par function_output double size=4; delta_t function_input double size=1; NotAus input boolean size=1; EinAus input boolean size=1; Richten input boolean size=1; ErrorSignal input boolean size=1; excute_signal input boolean size=1; Motor_status input boolean size=1; status output double size=1 =0; ZZP data_store_memory; ZZP_wait data_store_memory; parameter output double size=4; AP data_store_memory size=1; delta_T input double size=1
  function par = Par_1(delta_t):
    | function par = Par_1(delta_t)
    | 
    | global ZZP
    | global ZZP_wait
    | global AP
    | 
    | % delta_T = 10 s
    | ZZP = 0;
    | ZZP_wait = 0;
    | s0 = ZZP - AP;
    | a_max = 100;        % 1 m/s^2
    | v_max = 1;
    | %v_max = 0.5 * a_max * (delta_t - sqrt(delta_t*delta_t - 4*abs(s0)/a_max));   	% mm/s
    | 
    | par = [delta_t, a_max, v_max, s0]';
    | end
  function par = Par(delta_t):
    | function par = Par(delta_t)
    | 
    | global ZZP
    | global AP
    | 
    | s0 = ZZP - AP;
    | a_max = 1000;       % 1 m/s^2
    | v_max = 0.5 * a_max * (delta_t - sqrt(delta_t*delta_t - 4*abs(s0)/a_max));  % mm/s
    | 
    | par = [delta_t, a_max, v_max, s0]';
    | end

== matlab function Test_Agent_Motor/MotionSM_1/Motor/MATLAB Function1 ==
  settings: updateMethod=DISCRETE
  data: V output; v input; direction input double size=1; AP data_store_memory; ZZP data_store_memory
function V = v_conrol(v, direction)

global AP
global ZZP

if direction > 0
    if ((v < 0) || (AP >= ZZP))
        V = 0;
    else
        V = v;
    end
elseif direction < 0
    if v > 0 || (AP <= ZZP)
        V = 0;
    else
        V = v;
    end
else
    V = 0;
end
end

== matlab function Test_Agent_Motor/MotionSM_1/Motor/MATLAB Function2 ==
  settings: updateMethod=DISCRETE
  data: s input; s_old input; S output; direction input double size=1; AP data_store_memory; ZZP data_store_memory
function S = s_control(s, s_old, direction)

global AP
global ZZP

if direction > 0
    if (AP + s - s_old) < ZZP
        S = s;
        AP = AP + s - s_old;
    else
        S = s_old;
        AP = ZZP;
    end
elseif direction < 0
    if (AP + s - s_old) > ZZP
        S = s;
        AP = AP + s - s_old;
    else
        S = s_old;
        AP = ZZP;
    end
else
    S = s_old;
end

end

== stateflow chart Test_Agent_Motor/CommSM_1/Status_Control ==
  state Init
    entry: 	status=1;
    send_AT_package=[Adresse, zeros(1,5)];
    send_signal=false;
    send_MotionSM=[0,0];
  state Aus
    entry: status=0;
  state Ein
    state State_Control [parallel]
      settings: executionOrder=1
      note: % Protokoll
          | % SummenTelegramm = [HDR, SDT, END]
          | %HDR: header, SDT: Summen-Daten-Telegramm, END: Ender
          |
          | % SDT = [SDT_7, SDT_1, SDT_2, SDT_3]
          | % SDT_i = [Da_i, De_i]
          | %Da: Data, De: Delay
          | %i...{1,2,3,7} %7...GSM, 1-3...CommSM1-3
          |
          | % Da_i = [sender, receiver, cmd, N, ZP, ZP_status]
          | %sender,receiver...{1,2,3,7,255} %255...Broadcast
          | %cmd: 1...addP, 2...getP, 3...setS, 4...getS
          | %ZP_status: 0...none, 1...wait, 2...active, 3...done, 4...error
          |
          | % Da_i = [sender, receiver, cmd, N, s , s _status]
          | %cmd: 5 ...negO
          | % s _status: 0...none, 1...negotiation, 2...excute, 3...done
      note: 问题
          | 如何检测下一个新的ZP
      state send_AT_2_GSM
        entry:	status=16;
        permission=true;
        send_AT_package=[Adresse, 7, 3, ZPT_1(N,1:3)];
        %AT=[CommSM, GSM, setS, n, ZP, done];
        send_signal=true;
      state Free
        entry:	status=2;
      state Arrival
        entry:	status=15;
        ZPT_1(N,3)=3;
      state check_ZPT
        entry:	status=3;
        ZPT_1(N,3)=2;	      % status='active'
      state wait_arrival
        entry: status=14
      state send_Status_activ
        entry:	status=4;
        permission = true;
        send_AT_package = [Adresse, 7, 113, ZPT_1(N,1:3)];
        % AT=[CommSM, GSM, setS, n, ZP, activ];
        send_signal = true;
      state check_ZP
        entry: 	status=5;
        s=checkZP(ZZP_old, Adresse, N);
        % s-range: [0, 100], ZZP_old: ZZP for last loop
      state MotionSM
        entry:	status=13;
        send_MotionSM=[3, ZZPT_1(Adresse,2)];	%excute ZZP
        a = ZPT_1(N,2); b = ZZPT_1(Adresse,2);
      state send_nego_1
        entry: 	status=6;
        permission = true;
        send_AT_package=[Adresse, 255, 115, ZPT_1(N,1), s, 1];
        % AT=[CommSM, Broadcast, negO, n, s, nego];
        send_signal=true;
      state Nego_wait
        entry: 	status=7;
      state send_excu
        entry:	status=12;
        permission = true;
        send_AT_package = [Adresse, 255, 5, ZPT_1(N,1), ZZPT_1(Adresse, 4), 2];
        %AT=[CommSM, Broadcast, negO, n, s, excu];
        send_signal = true;
      state Wait_excution
        entry:	status=11;
        send_MotionSM=[1, ZZPT_1(Adresse,2)]; %set ZZP
      state s_Compair
        entry: 	status=8;
        s_new=s_compair(Adresse);
      state status_excution
        entry: 	status=10;
        ZZPT_1(Adresse,4)=2; %excu
      state ZZP_new
        entry:	status=9;
        ZZPT_1(Adresse,3)=s_new;
        ZZPT_1(Adresse,2)=AP+(ZPT_1(N,2)-AP)*(s_new/100);
      (default) -> Free
      send_AT_2_GSM -> Free : {send_signal=false; permission = false;}
      Free -> check_ZPT : % status ='wait' && MotionSM kein Fehler
          | [N>0 && ZPT_1(N,3)==1 && status_MotionSM>=1]{send_signal = false;}
      (junction 77) -> send_AT_2_GSM : [~permission]
      Arrival -> (junction 77)
      (junction 121) -> (junction 77)
      wait_arrival -> Arrival : % ZP == ZZP -> wait until ZP == AP
          | [isequal([ZPT_1(N,2), status_MotionSM],[AP, 2])]
          | {ZZPT_1=zeros(3,4);}
      check_ZPT -> send_Status_activ : [ZPT_1(N,3)==2 && ~permission]
      MotionSM -> wait_arrival [order 2] : % ZP == ZZP -> ZP will be arrived & no next ZP -> end
          | [status_MotionSM==3 && a==b && isempty(find(ZPT_1(:,3)==1,1))]
          | {send_MotionSM=zeros(1,2)}
      send_Status_activ -> (junction 99) : {send_signal = false; permission = false;}
      (junction 116) -> (junction 99)
      (junction 148) -> (junction 116)
      (junction 99) -> check_ZP
      MotionSM -> (junction 116) [order 1] : % ZP~=ZZP -> ZP will not be arrived -> negotiate again
          | [status_MotionSM==3 && a~=b]
          | {ZZP_old = ZZPT_1(Adresse,2); ZZPT_1 = zeros(3,4);}
      MotionSM -> (junction 148) [order 3] : [false]
          | % ZP = ZZP -> ZP will be arrived -> new ZP wait to negotiate -> loop
          | %[status_MotionSM==3 && a==b && ~isempty(find(ZPT_1(:,3)==1,1))]
          | %{ZZP_old = ZZPT_1(Adresse,2); ZZPT_1 = zeros(3,4)}
      check_ZP -> send_nego_1 : [~permission]
      (junction 146) -> MotionSM : % Motor stoped
          | [status_MotionSM==2]
      (junction 125) -> (junction 146) : % ZZP received from MotionSM
          | [isequal(data_from_MotionSM(1:2),[2,ZZPT_1(Adresse,2)])]
          | {ZZP_old=0;}
      send_excu -> (junction 125) : % all axis excuteable
          | [isequal(ZZPT_1(1:3,4),[2,2,2]')]
          | {send_signal=false; permission = false;}
      send_nego_1 -> Nego_wait : {s=0; send_signal=false; permission = false;}
      Nego_wait -> (junction 121) [order 1] : % ZP = AP, ZP schon erreicht
          | [ZPT_1(N,3)==3]
      Nego_wait -> (junction 134) [order 2] : % ZP~=AP, ZP "activ"
          | [ZPT_1(N,3)==2]
      Wait_excution -> send_excu : [~permission]
      (junction 134) -> s_Compair : % ob ZZPT komplett erfüllt
          | [isequal(ZZPT_1(1:3,1),[1,1,1]')]
      status_excution -> Wait_excution : [status_MotionSM>=2]  % 2 or 3
      s_Compair -> (junction 79)
      (junction 66) -> status_excution : {s_new=0;}
      (junction 79) -> (junction 66) [order 2] : [s_new>=ZZPT_1(Adresse,3)]
      (junction 79) -> ZZP_new [order 1] : [s_new<ZZPT_1(Adresse,3)]
      ZZP_new -> (junction 66)
    state Send [parallel]
      settings: executionOrder=2
      state wait
      state send
        entry: permission = true;
        send_AT_package = [Adresse, 7, 2, ZPT_1(n-1,1:3)];
        send_signal = true;
      (default) -> wait
      wait -> (junction 181) : % Requirement to respond GSM
          | [respond]
      (junction 186) -> wait : % send done
          | [~respond]{send_signal = false; permission = false;}
      (junction 181) -> send : % permission to use send_port
          | [~permission]
      send -> (junction 186) : [send_signal]{respond = false;}
  state Error
    entry: status=-1;
  (default) -> Aus
  Aus -> Init : [EinAus && ~NotAus && ~ErrorSignal]
  Init -> Aus [order 2] : [~EinAus]
  Init -> Error [order 3] : [NotAus]
  Error -> Aus [order 1] : [~EinAus]
  Ein -> Aus [order 1] : [~EinAus]
  Error -> Init [order 2] : [Richten && ~NotAus && ~ErrorSignal]
  Init -> Ein [order 1] : [status_Schnittstelle==4]{send_signal=false;}
  Ein -> Error [order 2] : [NotAus]
  data: zzp_old function_input double size=1; S function_output; adress function_input double size=1; N_ function_input; S_new function_output double size=1; nr function_input double size=1; Adresse input double size=1; status_Schnittstelle input double size=1; n input; N input; NotAus input boolean size=1; EinAus input boolean size=1; Richten input boolean size=1; ErrorSignal input boolean size=1; status output double size=1; send_signal output boolean size=1 =false; send_AT_package output double size=[1,6] =zeros(1,6); status_MotionSM input double size=1; data_from_MotionSM input double size=[1,2]; ZPT_1 data_store_memory; ZZPT_1 data_store_memory; AP data_store_memory; s local double size=1 =0; s_new local double size=1 =0; send_MotionSM output double size=[1,2] =zeros(1,2); ZZP_old local double size=1 =0; permission local boolean size=1 =false; respond data_store_memory; a local; b local
  function S = checkZP(zzp_old, adress, N_):
    | %ZPT_1 = [10x3], [ZP_Nr., ZP, status]
    | %status: {0...none, 1...wait, 2...active, 3...done, 4...error}
    | 
    | %ZZPT_1(CommSM_i,:) = [ZP-Nr., ZZP, s%, status]
    | %status: {0...none, 1...negotiation, 2...excution, 3...done}
    | 
    | function S = checkZP(zzp_old, adress, N_)
    | %1. prüfen, ob ZP unter begrenzte Bedienung erreichbar ist
    |         %Ja     --> ZZP = ZP
    |         %Nein   --> neuen ZZP erzeugen
    | %2. neu ausgerechnete ZZP in der ZZP Tabelle einschreiben
    |  
    | global AP
    | global ZPT_1
    | global ZZPT_1
    | 
    | a_max = 1000;   % mm/s^2
    | v_max = 1000;   % mm/s
    | d_T = 10;    % s
    | 
    | s_max = a_max*d_T*d_T/4;
    | if zzp_old <= 0             %last ZZP to arrive. After the Motor is started, ZZP_old = ZZP, ZZPT = zeros(3,4);
    |     s0 = ZPT_1(N_,2) - AP;     %ZP - AP
    | else
    |     s0 = ZPT_1(N_,2) - zzp_old;    %excist last ZZP
    | end
    | 
    | if abs(s0) <= s_max
    |     S = 100;                    % 100% erreichbar
    | elseif abs(s0) > 0 && abs(s0) < 100
    |     S = abs(100*s_max/s0);      % s% s: [0, 100]
    |     S = fix(1000*S)/1000;       % Genauigkeit = 10000*0.001%=0.1 mm
    | else
    |     S = 0;                      % ZP = AP, Achse keine Bewegung
    | end
    | 
    | %ZZP-Tabelle erfüllen
    | if zzp_old <= 0
    |     ZZP_new = AP + s0*S/100;        %neue ZZP in der ZZP-Tabelle einschreiben
    | else
    |     ZZP_new = zzp_old+s0*S/100;
    | end
    | 
    | if S == 0
    |     %ZZPT_1(nr,:) = [ZPT_1(1), ZZP_new, s, 3];
    |     ZPT_1(N_,3) = 3;
    | else
    |     ZZPT_1(adress,:) = [ZPT_1(N_,1), ZZP_new, S, 1];
    | end
    | 
    | end
  function S_new = s_compair(nr):
    | function S_new = s_compair(nr)
    | 
    | global ZZPT_1
    | 
    | s_ = ZZPT_1(:,3);
    | 
    | S_new = s_(nr);          % CommSM_me
    | 
    | for i = 1:3                         % s==0 --> s=100
    |     if i ~= nr && s_(i)== 0
    |         s_(i) = 100;
    |     end
    | end
    | 
    | s_min = min(s_);
    | if S_new > s_min
    |     S_new = s_min;
    | end
    | 
    | end

== matlab function Test_Agent_Motor/CommSM_1/MATLAB Function ==
  data: status input; n input; N input; signal input boolean size=1; package input double size=[1,7]; ZPT_1 data_store_memory; ZZPT_1 data_store_memory; respond data_store_memory
%Protokoll
%SummenTelegramm = [HDR, SDT, END]
	%HDR: header,	SDT: Summen-Daten-Telegramm,    END: Ender

%SDT = [SDT_7, SDT_1, SDT_2, SDT_3]
%SDT_i = [Da_i, De_i]
	%Da: Data, De: Delay
	%i...{1,2,3,7}	%7...GSM, 1-3...CommSM1-3

%Da_i = [sender, receiver, cmd, N, ZP, ZP_status]
	%sender,receiver...{1,2,3,7,255}	%255...Broadcast
	%cmd: 111...addP, 112...getP, 113...setS, 114...getS
	%ZP_status: 0...none, 1...wait, 2...active, 3...done, 4...error

%Da_i = [sender, receiver, cmd, N, s, s_status]
	%cmd: 115...negO
	%s_status: 0...none, 1...negotiation, 2...excute, 3...done


% Hier werden nur die Befehlen, die ZPT oder ZZPT ändern möchte, werden behandelt.
function receive_AT(status, n, N, signal, package)

% n - the first free row in ZPT_1 to add new ZP
% N - the line of currently handled ZP in ZPT_1

global ZPT_1
global ZZPT_1
global respond              % respond requirement, to let "send_AT" know, that it should answer the GSM

if (signal && (status >= 2))
    switch package(1)       % from GSM
        case 7
            switch package(3)
                case 111                    % cmd == 'add Position'
                    if (isempty(find(ZPT_1(:,1)==package(4),1)) && (n >= 1) && (n <= 10))
                        ZPT_1(n,:) = package(4:6)'; %[n, ZP, status='wait']
                        respond = true;
                    end
            end
            
        case {2,3}          % from CommSM_2 or CommSM_3
            switch package(3)
                case 115                    % negotiation
                    if ((N > 0) && (package(4) == ZPT_1(N,1)))
                        switch package(6)
                            case 1      % nego
                                if status == 7
                                    ZZPT_1(package(1),:) = [package(4), 0, package(5:6)];     % [n, ZP, s%, status='nego']
                                end
                            case 2      % excu
                                if ((status == 12) && (ZZPT_1(package(1),4) == 1))
                                    ZZPT_1(package(1),4) = package(6);                        % [n, ZP, s%, status='excu']
                                end
                        end
                    end
            end
    end
end

end

== matlab function Test_Agent_Motor/MATLAB Function ==
  data: u input; y output; u_old input
function y  = fcn(u,u_old)

if u_old
    y = false;
else
    y = u;
end
end
